simulink model "test3channel_c"  (Simulink 7.1)
settings: Solver=VariableStepDiscrete  StartTime=0.0  StopTime=0.0  RelTol=1e-3
libraries: SaliencyLib x1
settings Model: Creator=bruce  LastModifiedBy=bruce

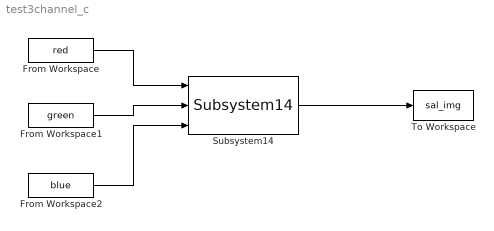
== system test3channel_c ==
  From Workspace : FromWorkspace  VariableName=red  SampleTime=0
  From Workspace1 : FromWorkspace  VariableName=green  SampleTime=0
  From Workspace2 : FromWorkspace  VariableName=blue  SampleTime=0
  Subsystem14 : SaliencyLib/Subsystem14  SystemSampleTime=-1  inRows=332  inCols=500
      link override Subsystem6/Subsystem17/Level-2 M-file S-Function: br=brxs  bc=bcxs
      link override Subsystem6/Subsystem17/Level-2 M-file S-Function5: br=brxs  bc=bcxs
      link override Subsystem6/Subsystem17/Level-2 M-file S-Function6: br=brxs  bc=bcxs
      link override Subsystem6/Subsystem17/Level-2 M-file S-Function7: br=brxs  bc=bcxs
  To Workspace : ToWorkspace  VariableName=sal_img  SampleTime=-1  SaveFormat=Structure
  wires:
  From Workspace/1 -> Subsystem14/1
  From Workspace1/1 -> Subsystem14/2
  From Workspace2/1 -> Subsystem14/3
  Subsystem14/1 -> To Workspace/1
